simulink model "parameter_tune"  (R2017b)
settings: Solver=FixedStepDiscrete  StartTime=0.0  StopTime=inf  RelTol=1e-3  EnableMultiTasking=on
InitFcn:
  | TuneGain = 1
libraries: pixhawk_slib_sensors_actuators x1
Description:
  | PX4 PSP Demo Model - parameter tune model
  | 
  | tuning parameters in external mode example
settings Model: SimulationMode=external  ExtModeBatchMode=on  TunableVars=TuneGain  TunableVarsStorageClass=Auto  Creator=skuznick  LastModifiedBy=skuznick
settings DataIOCC: LimitDataPoints=on  SaveFormat=Array  SignalLoggingSaveFormat=ModelDataLogs
settings OptimizationCC: DefaultParameterBehavior=Inlined  LifeSpan=1  MaxStackSize=64
settings DebuggingCC: SolverPrmCheckMsg=warning  MultiTaskDSMMsg=warning  MultiTaskCondExecSysMsg=none  AllowSymbolicDim=off  SFUnexpectedBacktrackingDiag=warning  SFNoUnconditionalDefaultTransitionDiag=warning  SFExecutionAtInitializationDiag=none
settings HardwareCC: ProdBitPerPointer=32  ProdBitPerSizeT=32  ProdBitPerPtrDiffT=32  ProdLargestAtomicInteger=Long  ProdLargestAtomicFloat=Double  ProdIntDivRoundTo=Undefined  ProdWordSize=32  ProdHWDeviceType=ARM Compatible->ARM Cortex
settings ModelReferenceCC: PropagateSignalLabelsOutOfModel=off
settings SFSimCC: MATLABDynamicMemAlloc=off
settings RTWCC: SystemTargetFile=ert.tlc  HardwareBoard=Pixhawk PX4  TLCOptions=-aInlineSetEventsForThisBaseRateFcn=TLC_FALSE -aSuppressMultiTaskScheduler=TLC_FALSE -aRateBasedStepFcn=0  TemplateMakefile=ert_default_tmf  GenerateReport=on  Toolchain=Pixhawk Toolchain  IncludeHyperlinkInReport=on  LaunchReport=on  GenerateTraceInfo=on  GenerateTraceReport=on  GenerateTraceReportSl=on  GenerateTraceReportSf=on  GenerateTraceReportEml=on  GenerateCodeMetricsReport=on
settings CodeAppCC: IgnoreCustomStorageClasses=off  StateflowObjectComments=on
settings ERTTargetCC: MultiwordLength=2048  ExtMode=on  ExtModeTransport=1  ExtModeStaticAllocSize=10000  ExtModeMexFile=ext_serial_win32_comm  ExtModeMexArgs=1 8 115200  ERTCustomFileTemplate=px4_codertarget_file_process.tlc  ConvertIfToSwitch=off  SuppressUnreachableDefaultCases=off
settings ConfigComp: CovMetricSettings=dw  CovHtmlReporting=on  CovSaveCumulativeToWorkspaceVar=on  CovSaveSingleToWorkspaceVar=on  CovExternalEMLEnable=off  CovSFcnEnable=off

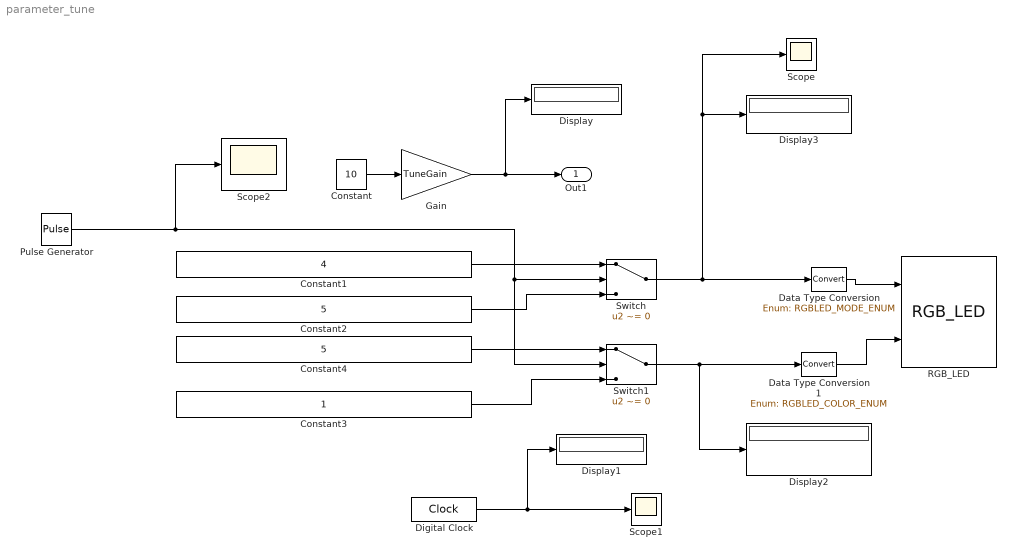
== system parameter_tune ==
  Constant : Constant  Value=10  SampleTime=0.1
  Constant1 : Constant  Value=4  OutDataTypeStr=int8
  Constant2 : Constant  Value=5  OutDataTypeStr=int8
  Constant3 : Constant  OutDataTypeStr=int8
  Constant4 : Constant  Value=5  OutDataTypeStr=int8
  Data Type Conversion : DataTypeConversion  OutDataTypeStr=Enum: RGBLED_MODE_ENUM
  Data Type Conversion1 : DataTypeConversion  OutDataTypeStr=Enum: RGBLED_COLOR_ENUM
  Digital Clock : DigitalClock  SampleTime=0.1
  Display{,1..3} (4 alike) : Display
  Gain : Gain  Gain=TuneGain
  Pulse Generator : DiscretePulseGenerator  PulseType=Time based  Period=6  PulseWidth=50
  RGB_LED : pixhawk_slib_sensors_actuators/RGB_LED
      settings: SourceProductName=Pixhawk Target Blocks
  Scope : Scope
  Scope1 : Scope
  Scope2 : Scope
  Switch : Switch  Criteria=u2 ~= 0  Threshold=1500
  Switch1 : Switch  Criteria=u2 ~= 0  Threshold=1500
  Out1 : Outport
  wires:
  Constant/1 -> Gain/1
  Gain/1 -> Display/1, Out1/1
  Switch/1 -> Scope/1, Display3/1, Data Type Conversion/1
  Switch1/1 -> Display2/1, Data Type Conversion1/1
  Constant1/1 -> Switch/1
  Constant2/1 -> Switch/3
  Constant4/1 -> Switch1/1
  Constant3/1 -> Switch1/3
  Pulse Generator/1 -> Scope2/1, Switch1/2, Switch/2
  Digital Clock/1 -> Display1/1, Scope1/1
  Data Type Conversion/1 -> RGB_LED/1
  Data Type Conversion1/1 -> RGB_LED/2
